simulink model "basic_eqution"  (R2021a)
settings: Solver=VariableStepAuto  StartTime=0.0  StopTime=10.0  RelTol=1e-3
InitFcn:
  | x=10
settings Model: Creator=DELL  LastModifiedBy=DELL

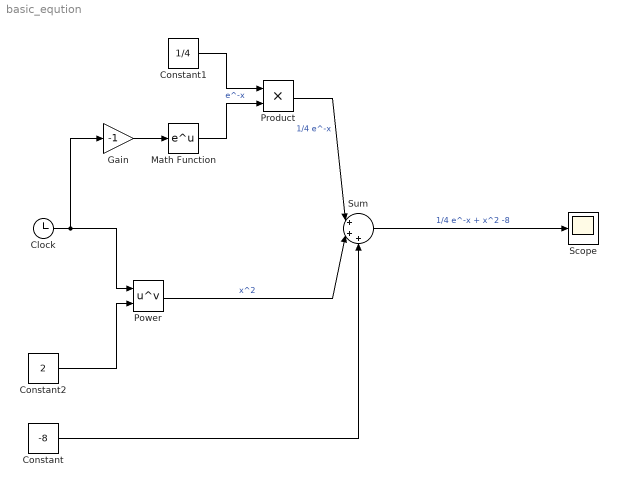
== system basic_eqution ==
  Clock : Clock
  Constant : Constant  Value=-8
  Constant1 : Constant  Value=1/4
  Constant2 : Constant  Value=2
  Gain : Gain  Gain=-1
  Math Function : Math  SaturateOnIntegerOverflow=on
  Power : Math  Operator=pow  SaturateOnIntegerOverflow=on
  Product : Product
  Scope : Scope
  Sum : Sum  Inputs=|+++
  wires:
  Math Function/1 -> Product/2  "e^-x"
  Constant1/1 -> Product/1
  Constant2/1 -> Power/2
  Clock/1 -> Gain/1, Power/1
  Product/1 -> Sum/1  "1/4 e^-x"
  Power/1 -> Sum/2  "x^2"
  Constant/1 -> Sum/3
  Sum/1 -> Scope/1  "1/4 e^-x + x^2 -8"
  Gain/1 -> Math Function/1
